simulink library "mpc555drivers"  (Simulink 6.0)
settings: Solver=ode45  SolverMode=SingleTasking  StartTime=0.0  StopTime=10.0  RelTol=1e-3
PreLoadFcn:
  | RTWConfigurationCB('preloadfcn', bdroot);
InitFcn:
  | % START RTW CONFIGURATION CODE %
  | RTWConfigurationCB('rtw_target_initfcn',gcs);
  | % END RTW CONFIGURATION CODE %
undefined symbols (not defined in the file or in its folder): pmax, scale
libraries: passthrough x52, driver_interface_library x18, mpc555toucan x11, mpc555extras x9, config_library x7, exprofilelib x4, simulink x3, mpc555drivers x2, canblocks x1
(part 2 of 3)

== system mpc555drivers/Time Processor Unit (TPU3) ==
  Subsystem Resource Configuration Class : config_library/Subsystem Resource Configuration Class  Tag=CONFIGURATION DATA CLASS  dClassName=MPC555dkConfig.TPU  rClassName=MPC555dkConfig.TPU_RESOURCES
  TPU3 Digital In : Subsystem  PropExecContextAcrossSSBoundary=on  mask(MPC555 Digital Input (TPU3)){module=A, channel=0, channel_priority=Medium, sampleTime=0.1, enablePassThru=off}
      mask prompts: module "TPU module:"; channel "TPU channel number:"; channel_priority "Channel priority:"; sampleTime "Sample time:"; enablePassThru "Enable pass through (show simulation input)"
      mask help: Configures a Time Processor Unit (TPU3) channel for digital input. Reads the logical state of the specified TPU channel pin.
      mask init:
      | simulinkPortControl(gcbh,'enable','PassThrough',enablePassThru);
      | 
      | %Deprecation warning for passthrough
      | if (enablePassThru)
      | 	passThroughDeprecationWarning;
      | end;
      | 
      | % decrement the channel to map from 0..15
      | channel = channel - 1;
      | 
      | % verify module selection
      | mpc5xx_tpu_verify_modules(gcb);
      | 
      | % Perform Resource Configuration
      | type = ['TPU_' module '_CHANNELS'];
      | RTWConfiguration.Target.acquireResourceForBlock(      ...
      |    gcb,                    ...   % Current block
      |    'MPC555dkConfig.TPU', ...   % Configuration Class
      |    type,          ...   % Resource Type associated with the configuration class
      |    num2str(channel),                    ...   % Resource being requested
      |    'TPU Channel'            ...   % Lable to be used in error messages
      | );
      mask Help: helpview([docroot '/toolbox/mpc555dk/mpc555dk.map'], 'TPU_Dig_In');
      mask StyleString: popup(A|B|C),popup(0|1|2|3|4|5|6|7|8|9|10|11|12|13|14|15),popup(Low|Medium|High),edit,checkbox
      mask Display: disp(['Digital In\n(TPU3)']);
  TPU3 Digital Out : Subsystem  PropExecContextAcrossSSBoundary=on  mask(MPC555 Digital Output (TPU3)){module=A, channel=0, channel_priority=Medium, sampleTime=-1, enablePassThru=off}
      mask prompts: module "TPU module:"; channel "TPU channel number:"; channel_priority "Channel priority:"; sampleTime "Sample time:"; enablePassThru "Enable pass through (show simulation output)"
      mask help: Configures a Time Processor Unit (TPU3) channel for digital output. When the input signal is greater than zero a logical one is written to the corresponding pin; otherwise a logical zero is written.
      mask init:
      | simulinkPortControl(gcbh,'enable','PassThrough',enablePassThru);
      | 
      | %Deprecation warning for passthrough
      | if (enablePassThru)
      | 	passThroughDeprecationWarning;
      | end;
      | 
      | % decrement the channel to map from 0..15
      | channel = channel - 1;
      | 
      | % verify module selection
      | mpc5xx_tpu_verify_modules(gcb);
      | 
      | % Perform Resource Configuration
      | type = ['TPU_' module '_CHANNELS'];
      | RTWConfiguration.Target.acquireResourceForBlock(      ...
      |    gcb,                    ...   % Current block
      |    'MPC555dkConfig.TPU', ...   % Configuration Class
      |    type,          ...   % Resource Type associated with the configuration class
      |    num2str(channel),                    ...   % Resource being requested
      |    'TPU Channel'            ...   % Lable to be used in error messages
      | );
      mask Help: helpview([docroot '/toolbox/mpc555dk/mpc555dk.map'], 'TPU_Dig_Out');
      mask StyleString: popup(A|B|C),popup(0|1|2|3|4|5|6|7|8|9|10|11|12|13|14|15),popup(Low|Medium|High),edit,checkbox
      mask Display: disp(['Digital Out\n (TPU3)'])
  TPU3 Fast Quadrature Decode : Subsystem  PropExecContextAcrossSSBoundary=on  mask(MPC555 Fast Quadrature Decode (TPU3)){module=A, channel=0 and 1, channel_priority=Medium, fast_mode=off, init_position_count=0, pc_alias=, sampleTime=0.1, enablePassThru=off}
      mask prompts: module "TPU module:"; channel "TPU channel numbers (primary and secondary):"; channel_priority "Channel priority:"; fast_mode "Show Fast Mode port"; init_position_count "Initial value for POSITION_COUNT:"; pc_alias "POSITION_COUNT parameter alias (optional):"; sampleTime "Sample time:"; enablePassThru "Enable pass through (show simulation input)"
      mask help:
      | Configures a pair of Time Processor Unit (TPU3) channels for Fast Quadrature Decode (FQD).   Decodes a pair of out-of-phase input signals in order to increment or decrement the position counter (block output).
      |
      | The POSITION_COUNT parameter can be made available easily to other TPU blocks such as the NITC function by providing an alias.
      mask init:
      | % enable / disable ports according to mask selections
      | simulinkPortControl(gcbh, 'enable', 'FastMode', fast_mode);
      | simulinkPortControl(gcbh, 'enable', 'PassThrough', enablePassThru);
      | 
      | %Deprecation warning for passthrough
      | if (enablePassThru)
      | 	passThroughDeprecationWarning;
      | end;
      | 
      | % decrement the channel to map from 0..15
      | channel = channel - 1;
      | % resource allocation for the primary channel + secondary channel
      | % mpc555_tpu_fqd_validate acquires resouce for primary channel, and
      | % primary channel + 1 (secondary channel)
      | % Perform Resource Configuration
      | type = ['TPU_' module '_CHANNELS'];
      | 
      | % verify module selection
      | mpc5xx_tpu_verify_modules(gcb);
      | 
      | RTWConfiguration.Target.acquireResourceForBlock(      ...
      |    gcb,                    ...   % Current block
      |    'MPC555dkConfig.TPU', ...   % Configuration Class
      |    type,          ...   % Resource Type associated with the configuration class
      |    { num2str(channel) num2str(channel+1) },                    ...   % Resource being requested
      |    'TPU Channel'            ...   % Lable to be used in error messages
      | );
      | 
      | % make sure the variables are consistent
      | % we cannot just rely on the mask callbacks!
      | mpc555_tpu_fqd_config('model_initialisation', gcb, init_position_count);
      mask Help: helpview([docroot '/toolbox/mpc555dk/mpc555dk.map'], 'TPU_Fast_Quad_Decode');
      mask StyleString: popup(A|B|C),popup(0 and 1|1 and 2|2 and 3|3 and 4|4 and 5|5 and 6|6 and 7|7 and 8|8 and 9|9 and 10|10 and 11|11 and 12|12 and 13|13 and 14|14 and 15),popup(Low|Medium|High),checkbox,edit,edit,edit,checkbox
      mask CallbackString: ||||mpc555_tpu_fqd_config('initPositionCallback', gcbh);|||
      mask Display: disp(sprintf('FQD\n(TPU3)'));
  TPU3 New Input Capture/ Input Transition Counter : Subsystem  PropExecContextAcrossSSBoundary=on  mask(MPC555 New Input Capture/Input Transition Counter (TPU3)){module=A, channel=0, channel_priority=Medium, finalTransTime=on, transCount=off, lastTransTime=off, transitionType=Rising Edge, captureType=TCR1 Value, parameterLocation=Channel and Parameter Index, captureChannel=0, captureParam=0, captureParamAlias=, maxCount=1, sampleTime=0.1, enablePassThru=off}
      mask prompts: module "TPU module:"; channel "TPU channel number:"; channel_priority "Channel priority:"; finalTransTime "Show FINAL_TRANS_TIME port"; transCount "Show TRANS_COUNT port"; lastTransTime "Show LAST_TRANS_TIME port"; transitionType "Detect transition on:"; captureType "Capture:"; parameterLocation "Specify parameter location by:"; captureChannel "TPU channel to capture parameter from:"; captureParam "Channel parameter (16-bit) to capture:"; captureParamAlias "Parameter alias:"; maxCount "Number of transitions before capture and reset (MAX_COUNT):"; sampleTime "Sample time:"; enablePassThru "Enable pass through  (show simulation input)"
      mask help: Configures a Time Processor Unit (TPU3) channel for New Input Capture/Input Transition Counter (NITC). Counts individual transitions on the input pin, and allows the capture of a TCR or TPU parameter RAM value after a selectable number of pin transitions.
      mask init:
      | % enable / disable ports according to mask selections
      | simulinkPortControl(gcbh, 'enable', 'FinalTransTime', finalTransTime);
      | simulinkPortControl(gcbh, 'enable', 'TransCount', transCount);
      | simulinkPortControl(gcbh, 'enable', 'LastTransTime', lastTransTime);
      | simulinkPortControl(gcbh, 'enable', 'PassThroughFinalTransTime', finalTransTime & enablePassThru);
      | simulinkPortControl(gcbh, 'enable', 'PassThroughTransCount', transCount & enablePassThru);
      | simulinkPortControl(gcbh, 'enable', 'PassThroughLastTransTime', lastTransTime & enablePassThru);
      | 
      | %Deprecation warning for passthrough
      | if (enablePassThru)
      | 	passThroughDeprecationWarning;
      | end;
      | 
      | % decrement the channel to map from 0..15
      | channel = channel - 1;
      | % decrement the capture channel to map from 0..15
      | captureChannel = captureChannel - 1;
      | % decrement the capture param to map from 0..7
      | captureParam = captureParam - 1;
      | 
      | % check the MAX_COUNT param at model update time
      | % as well as in the mask callback
      | mpc555_tpu_nitc_config('model_initialisation', gcb, maxCount);
      | 
      | % check the alias parameter is not empty
      | if captureType == 2 && parameterLocation == 2
      | 	captureParamAlias = strtrim(captureParamAlias);
      | 	if isempty(captureParamAlias)
      | 		error(sprintf('\n"Named parameter to be captured" parameter cannot be empty'));
      | 	end
      | end
      | 
      | % verify module selection
      | mpc5xx_tpu_verify_modules(gcb);
      | 
      | % Perform Resource Configuration
      | type = ['TPU_' module '_CHANNELS'];
      | RTWConfiguration.Target.acquireResourceForBlock(      ...
      |    gcb,                    ...   % Current block
      |    'MPC555dkConfig.TPU', ...   % Configuration Class
      |    type,          ...   % Resource Type associated with the configuration class
      |    num2str(channel),                    ...   % Resource being requested
      |    'TPU Channel'            ...   % Lable to be used in error messages
      | );
      mask Help: helpview([docroot '/toolbox/mpc555dk/mpc555dk.map'], 'TPU_NITC');
      mask StyleString: popup(A|B|C),popup(0|1|2|3|4|5|6|7|8|9|10|11|12|13|14|15),popup(Low|Medium|High),checkbox,checkbox,checkbox,popup(Rising Edge|Falling Edge|Either Edge),popup(TCR1 Value|Parameter RAM Value),popup(Channel and Parameter Index|Parameter Alias),popup(0|1|2|3|4|5|6|7|8|9|10|11|12|13|14|15),popup(0|1|2|3|4|5|6|7),edit,edit,edit,checkbox
      mask CallbackString:
      | |||||||switch get_param(gcb,'captureType')
      | 	case 'TCR1 Value'
      | 	    simUtil_maskParam('disable', gcb, 'parameterLocation');
      | 	case 'Parameter RAM Value'
      | 		simUtil_maskParam('enable', gcb, 'parameterLocation');
      | end
      | simUtil_maskParam('execcallback', gcb, 'parameterLocation');|if simUtil_maskParam('isenable', gcb, 'parameterLocation')
      | 	switch get_param(gcb,'parameterLocation')
      | 	case 'Channel and Parameter Index'
      | 	    simUtil_maskParam('enable', gcb, 'captureChannel');
      | 		simUtil_maskParam('enable', gcb, 'captureParam');
      | 		simUtil_maskParam('disable', gcb, 'captureParamAlias');
      | 
      | 	case 'Parameter Alias'
      | 		simUtil_maskParam('disable', gcb, 'captureChannel');
      | 		simUtil_maskParam('disable', gcb, 'captureParam');
      | 		simUtil_maskParam('enable', gcb, 'captureParamAlias');
      | 	end
      | else
      | 		simUtil_maskParam('disable', gcb, 'captureChannel');
      | 		simUtil_maskParam('disable', gcb, 'captureParam');
      | 		simUtil_maskParam('disable', gcb, 'captureParamAlias');
      | end||||mpc555_tpu_nitc_config('max_count_callback', gcb);||
      mask Display: disp(['NITC\n(TPU3)']);
  TPU3 Programmable Time Accumulator : Subsystem  PropExecContextAcrossSSBoundary=on  mask(MPC555 Programmable Time Accumulator (TPU3)){module=A, channel=0, channel_priority=Medium, timeAccum=on, periodCount=off, mode=Total high time, maxCount=1, sampleTime=0.1, enablePassThru=off}
      mask prompts: module "TPU module:"; channel "TPU channel number:"; channel_priority "Channel priority:"; timeAccum "Show time accumulation (32-bit) port"; periodCount "Show PERIOD_COUNT port"; mode "Measure:"; maxCount "Number of periods to measure over (MAX_COUNT):"; sampleTime "Sample time:"; enablePassThru "Enable pass through (show simulation input)"
      mask help: Configures a Time Processor Unit (TPU3) channel for Programmable Time Accumulator (PTA). Measures high time, low time or total period over a selectable number of periods on the input pin.
      mask init:
      | % enable / disable ports according to mask selections
      | simulinkPortControl(gcbh, 'enable', 'TimeAccum', timeAccum);
      | simulinkPortControl(gcbh, 'enable', 'PeriodCount', periodCount);
      | simulinkPortControl(gcbh, 'enable', 'PassThroughTimeAccum', timeAccum & enablePassThru);
      | simulinkPortControl(gcbh, 'enable', 'PassThroughPeriodCount', periodCount & enablePassThru);
      | 
      | %Deprecation warning for passthrough
      | if (enablePassThru)
      | 	passThroughDeprecationWarning;
      | end;
      | 
      | % decrement the channel to map from 0..15
      | channel = channel - 1;
      | 
      | % check the MAX_COUNT param at model update time
      | % as well as in the mask callback
      | mpc555_tpu_pta_config('model_initialisation', gcb, maxCount);
      | 
      | % verify module selection
      | mpc5xx_tpu_verify_modules(gcb);
      | 
      | % Perform Resource Configuration
      | type = ['TPU_' module '_CHANNELS'];
      | RTWConfiguration.Target.acquireResourceForBlock(      ...
      |    gcb,                    ...   % Current block
      |    'MPC555dkConfig.TPU', ...   % Configuration Class
      |    type,          ...   % Resource Type associated with the configuration class
      |    num2str(channel),                    ...   % Resource being requested
      |    'TPU Channel'            ...   % Lable to be used in error messages
      | );
      mask Help: helpview([docroot '/toolbox/mpc555dk/mpc555dk.map'], 'TPU_PTA');
      mask StyleString: popup(A|B|C),popup(0|1|2|3|4|5|6|7|8|9|10|11|12|13|14|15),popup(Low|Medium|High),checkbox,checkbox,popup(Total high time|Total low time|Total period (start on rising edge)|Total period (start on falling edge)),edit,edit,checkbox
      mask CallbackString: ||||||mpc555_tpu_pta_config('max_count_callback', gcb);||
      mask Display: disp(['PTA\n(TPU3)']);
  TPU3 Pulse Width Modulation Out : Subsystem  PropExecContextAcrossSSBoundary=on  mask(MPC555 Pulse Width Modulation Output (TPU3)){module=A, channel=0, channel_priority=Medium, block_period=off, timing_settings=off, ideal_period=0.02, PWMPER=12500, actual_period=0.02, sampleTime=-1, enablePassThru=off}
      mask prompts: module "TPU module:"; channel "TPU channel number:"; channel_priority "Channel priority:"; block_period "Use input port for pulse period register value"; timing_settings "Edit period register manually"; ideal_period "Waveform ideal period:"; PWMPER "Pulse period register (PWMPER):"; actual_period "Waveform actual period:"; sampleTime "Sample time:"; enablePassThru "Enable pass through (show simulation output)"
      mask help: Configures a Time Processor Unit (TPU3) channel for pulse width modulation (PWM) output. An input signal in the range 0 to 1 generates a PWM output with corresponding duty cycle; input signals above (below) this range cause the duty cycle to saturate at 100% (0%).
      mask init:
      | % enable / disable ports according to mask selections
      | simulinkPortControl(gcbh, 'enable', 'Period', block_period);
      | simulinkPortControl(gcbh, 'enable', 'PassThroughDutyCycle', enablePassThru);
      | simulinkPortControl(gcbh, 'enable', 'PassThroughPeriod', enablePassThru & block_period);
      | 
      | %Deprecation warning for passthrough
      | if (enablePassThru)
      | 	passThroughDeprecationWarning;
      | end;
      | 
      | % decrement the channel to map from 0..15
      | channel = channel - 1;
      | 
      | % verify module selection
      | mpc5xx_tpu_verify_modules(gcb);
      | 
      | % Perform Resource Configuration
      | type = ['TPU_' module '_CHANNELS'];
      | RTWConfiguration.Target.acquireResourceForBlock(      ...
      |    gcb,                    ...   % Current block
      |    'MPC555dkConfig.TPU', ...   % Configuration Class
      |    type,          ...   % Resource Type associated with the configuration class
      |    num2str(channel),                    ...   % Resource being requested
      |    'TPU Channel'            ...   % Lable to be used in error messages
      | );
      | 
      | % make sure the variables are consistent
      | % we cannot just rely on the mask callbacks!
      | PWMPER = mpc555_tpu_pwm_config('model_initialisation',gcb, PWMPER, ideal_period);
      mask Help: helpview([docroot '/toolbox/mpc555dk/mpc555dk.map'], 'TPU_PWM_Out');
      mask StyleString: popup(A|B|C),popup(0|1|2|3|4|5|6|7|8|9|10|11|12|13|14|15),popup(Low|Medium|High),checkbox,checkbox,edit,edit,edit,edit,checkbox
      mask CallbackString: |||mpc555_tpu_pwm_config('block_period_callback',gcb);|mpc555_tpu_pwm_config('timing_settings_callback',gcb);|mpc555_tpu_pwm_config('ideal_period_callback',gcb);|mpc555_tpu_pwm_config('PWMPER_callback',gcb);|||
      mask Display: disp(sprintf('PWM Out\n(TPU3)'))

== system mpc555drivers/Watchdog ==
  Initialize Watchdog : mpc555extras/Custom Code  unique=Generate for every instance  key='_WATCHDOG_'  location=Model Start Function  top=''  middle=''  bottom=model_init_function_code

== system mpc555drivers/Enhanced Queued Analog-To-Digital Converter Module-64/QADCE Analog In ==
  note: NOTE: Data direction register has 0 reset value
      | ->
      | all pins configured for input
  Extended Custom Code : driver_interface_library/Custom Code
  RTW memory get : driver_interface_library/Input Driver  t=t  expr=register  portWidth=length(channels)  pOpt=[]  expression_type=Expression
  Subsystem : Subsystem  PropExecContextAcrossSSBoundary=on  mask{type=outDType}
      mask prompts: type "Data Type"
      mask init:
      | block = find_system(gcb,'followlinks','on','lookundermasks','on','tag','type_block');
      | set_param(block{1},'DataType',type);
  Out : Outport
  wires:
  Subsystem/1(Out1) -> Out/1
  RTW memory get/1 -> Subsystem/1(In1)

== system mpc555drivers/Enhanced Queued Analog-To-Digital Converter Module-64/QADCE Digital In ==
  note: NOTE: Data direction register has 0 reset value
      | ->
      | all pins configured for input
  Bitwise Operator1 : mpc555extras/Bitwise Operator  logicop=AND  zeroTest=Test If Not Zero  UseBitMask=on  BitMask=masks  maskInBinary=off
  Data Type Conversion : DataTypeConversion  OutDataTypeMode=boolean  SaturateOnIntegerOverflow=on  RndMeth=Zero
  RTW memory get : driver_interface_library/Input Driver  t=t  expr=register  portWidth=1  pOpt=[]  expression_type=Expression
  Signal Specification : SignalSpecification  DataType=uint8
  Out : Outport
  wires:
  Data Type Conversion/1 -> Out/1
  Signal Specification/1 -> Bitwise Operator1/1
  RTW memory get/1 -> Signal Specification/1
  Bitwise Operator1/1 -> Data Type Conversion/1

== system mpc555drivers/Execution Profiling/MPC555 Execution Profiling via CAN A ==
  Execution Profiling Output Data1 : exprofilelib/Execution Profiling Output Data  t=t
  Send data over CAN : Subsystem  TreatAsAtomicUnit=on  PropExecContextAcrossSSBoundary=on
  Start execution profiling : Subsystem  PropExecContextAcrossSSBoundary=on
  Terminator : Terminator
  TouCAN Receive : mpc555toucan/TouCAN Receive  module=A  ids=commandId  notification_type=Function Call Outport  auto_select_buffer=on  bufferids=14  use_queue=off  queue_length=3  message_type=Extended (29-bit identifier)  t=t
  wires:
  Execution Profiling Output Data1/2 -> Send data over CAN/1(In1)
  Execution Profiling Output Data1/1 -> Send data over CAN/Enable
  TouCAN Receive/1 -> Start execution profiling/Trigger
  TouCAN Receive/2 -> Terminator/1

== system mpc555drivers/Execution Profiling/MPC555 Execution Profiling via SCI1 ==
  Constant : Constant  OutDataTypeMode=uint32
  Send Execution Profiling Data via Serial : Subsystem  PropExecContextAcrossSSBoundary=on
  Serial Receive : mpc555drivers/Serial Communications Interface (SCI)/Serial Receive  module=1  show_length=on  max_length=1  show_reset=off  show_bytes_read=on  show_flags=off  show_overrun=off  T=t
  Serial Transmit Status : S-Function  FunctionName=qsmcm_sci_status  Parameters=T, module  mask(SCI Status){module=1, T=t}
      mask prompts: module "SCI module:"; T "Sample time:"
      mask help: Read data from the QSMCM SCI status register. In particular, the Transmission Complete flag TC is equal to 0 if a transmission is in progress, or 1 if any transmission is complete.
      mask init:
      | % check for a Resource Config block, and make sure it is MPC555
      | target = RTWConfigurationCB('get_target', gcb);
      | target.checkName('MPC555');
      mask StyleString: popup(1|2),edit
      mask Display: text(0.5, 0.5, ['SCI' num2str(module) '\nStatus'],'horizontalAlignment','center'); port_label('input',1,'Data'); port_label('output', 1, 'TC');
  Start Profiling : Subsystem  PropExecContextAcrossSSBoundary=on
  wires:
  Serial Transmit Status/1 -> Send Execution Profiling Data via Serial/Enable
  Constant/1 -> Serial Receive/1
  Serial Receive/1 -> Start Profiling/1(Data In)
  Serial Receive/2 -> Start Profiling/Enable  "num bytes received"

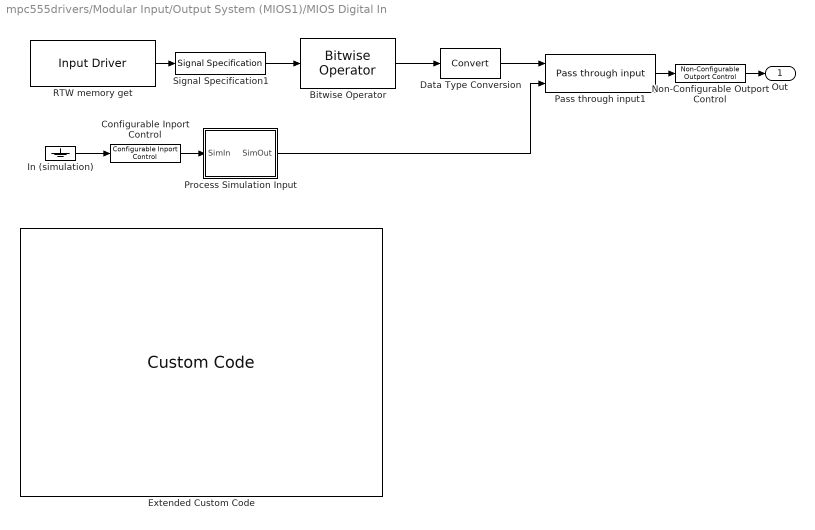
== system mpc555drivers/Modular Input/Output System (MIOS1)/MIOS Digital In ==
  Bitwise Operator : mpc555extras/Bitwise Operator  logicop=AND  zeroTest=No Test  UseBitMask=on  BitMask=masks  maskInBinary=on
  Configurable Inport Control : passthrough/Configurable Inport Control  portNum=1  portName=PassThrough  isEnabled=0  isConfigurable=1  isInport=1
  Data Type Conversion : DataTypeConversion  OutDataTypeMode=boolean  SaturateOnIntegerOverflow=on  RndMeth=Zero
  Extended Custom Code : driver_interface_library/Custom Code
  In (simulation) : Ground
  Non-Configurable Outport Control : passthrough/Non-Configurable Outport Control  portNum=1  isEnabled=1  isConfigurable=0  isInport=0
  Pass through input1 : passthrough/Pass through input
  Process Simulation Input : Subsystem  PropExecContextAcrossSSBoundary=on
  RTW memory get : driver_interface_library/Input Driver  t=t  expr='MIOS1.MPIOSM32DR.R'  portWidth=1  pOpt=[]  expression_type=Not expression
  Signal Specification1 : SignalSpecification  DataType=uint16
  Out : Outport
  wires:
  Pass through input1/1 -> Non-Configurable Outport Control/1
  RTW memory get/1 -> Signal Specification1/1
  In (simulation)/1 -> Configurable Inport Control/1
  Process Simulation Input/1(SimOut) -> Pass through input1/2
  Signal Specification1/1 -> Bitwise Operator/1
  Bitwise Operator/1 -> Data Type Conversion/1
  Data Type Conversion/1 -> Pass through input1/1
  Configurable Inport Control/1 -> Process Simulation Input/1(SimIn)
  Non-Configurable Outport Control/1 -> Out/1

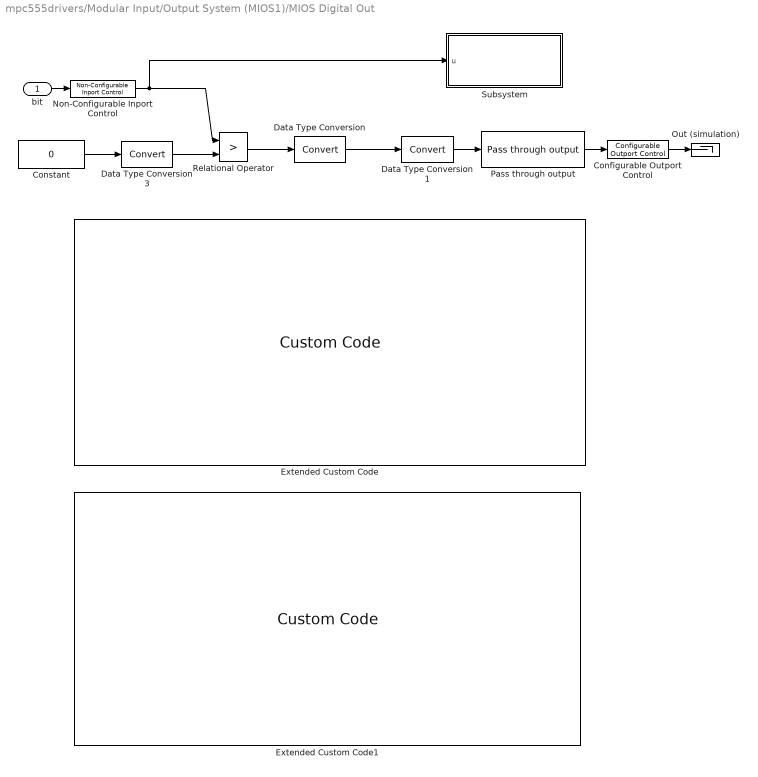
== system mpc555drivers/Modular Input/Output System (MIOS1)/MIOS Digital Out ==
  bit : Inport  Port=1  SampleTime=t  LatchInput=off
  Configurable Outport Control : passthrough/Configurable Outport Control  portNum=1  portName=PassThrough  isEnabled=0  isConfigurable=1  isInport=0
  Constant : Constant  Value=0
  Data Type Conversion : DataTypeConversion  OutDataTypeMode=boolean  SaturateOnIntegerOverflow=on  RndMeth=Zero
  Data Type Conversion1 : DataTypeConversion  SaturateOnIntegerOverflow=on  RndMeth=Zero
  Data Type Conversion3 : DataTypeConversion  SaturateOnIntegerOverflow=on  RndMeth=Zero
  Extended Custom Code : driver_interface_library/Custom Code
  Extended Custom Code1 : driver_interface_library/Custom Code
  Non-Configurable Inport Control : passthrough/Non-Configurable Inport Control  portNum=1  isEnabled=1  isConfigurable=0  isInport=1
  Out (simulation) : Terminator
  Pass through output : passthrough/Pass through output  driverBlock=gcs
  Relational Operator : RelationalOperator  Operator=>  InputSameDT=on
  Subsystem : Subsystem  TreatAsAtomicUnit=on  PropExecContextAcrossSSBoundary=on
  wires:
  bit/1 -> Non-Configurable Inport Control/1
  Relational Operator/1 -> Data Type Conversion/1
  Constant/1 -> Data Type Conversion3/1
  Data Type Conversion/1 -> Data Type Conversion1/1
  Pass through output/1 -> Configurable Outport Control/1
  Data Type Conversion1/1 -> Pass through output/1
  Data Type Conversion3/1 -> Relational Operator/2
  Non-Configurable Inport Control/1 -> Relational Operator/1, Subsystem/1(u)
  Configurable Outport Control/1 -> Out (simulation)/1

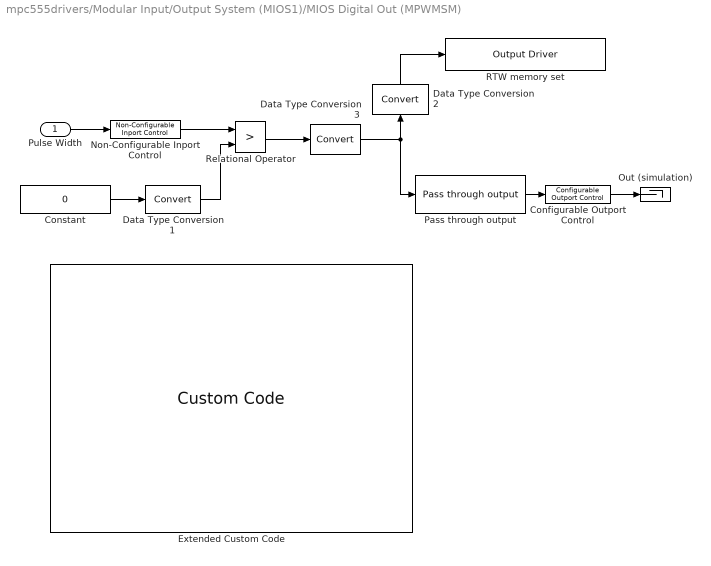
== system mpc555drivers/Modular Input/Output System (MIOS1)/MIOS Digital Out (MPWMSM) ==
  Pulse Width : Inport  Port=1  LatchInput=off
  Configurable Outport Control : passthrough/Configurable Outport Control  portNum=1  portName=PassThrough  isEnabled=0  isConfigurable=1  isInport=0
  Constant : Constant  Value=0
  Data Type Conversion1 : DataTypeConversion  SaturateOnIntegerOverflow=on  RndMeth=Zero
  Data Type Conversion2 : DataTypeConversion  Orientation=up  OutDataTypeMode=uint16  SaturateOnIntegerOverflow=on  RndMeth=Zero
  Data Type Conversion3 : DataTypeConversion  SaturateOnIntegerOverflow=on  RndMeth=Zero
  Extended Custom Code : driver_interface_library/Custom Code
  Non-Configurable Inport Control : passthrough/Non-Configurable Inport Control  portNum=1  isEnabled=1  isConfigurable=0  isInport=1
  Out (simulation) : Terminator
  Pass through output : passthrough/Pass through output  driverBlock=gcs
  RTW memory set : driver_interface_library/Output Driver  operation_type=LHS Assignment  input_is_contiguous=off  t=t  expr=[ 'MIOS1.MPWMSM' module 'SCR.B.POL']  port_width=1  pOpt=[]
  Relational Operator : RelationalOperator  Operator=>  InputSameDT=on
  wires:
  Pass through output/1 -> Configurable Outport Control/1
  Pulse Width/1 -> Non-Configurable Inport Control/1
  Relational Operator/1 -> Data Type Conversion3/1
  Constant/1 -> Data Type Conversion1/1
  Data Type Conversion1/1 -> Relational Operator/2
  Data Type Conversion2/1 -> RTW memory set/1
  Data Type Conversion3/1 -> Data Type Conversion2/1, Pass through output/1
  Non-Configurable Inport Control/1 -> Relational Operator/1
  Configurable Outport Control/1 -> Out (simulation)/1

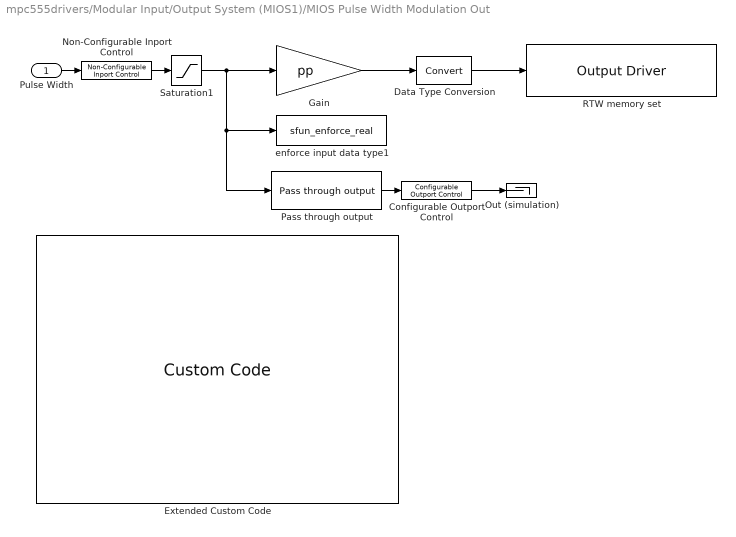
== system mpc555drivers/Modular Input/Output System (MIOS1)/MIOS Pulse Width Modulation Out ==
  Pulse Width : Inport  Port=1  SampleTime=t  LatchInput=off
  Configurable Outport Control : passthrough/Configurable Outport Control  portNum=1  portName=PassThrough  isEnabled=0  isConfigurable=1  isInport=0
  Data Type Conversion : DataTypeConversion  OutDataTypeMode=uint16  RndMeth=Zero
  Extended Custom Code : driver_interface_library/Custom Code
  Gain : Gain  Gain=pp  SaturateOnIntegerOverflow=on
  Non-Configurable Inport Control : passthrough/Non-Configurable Inport Control  portNum=1  isEnabled=1  isConfigurable=0  isInport=1
  Out (simulation) : Terminator
  Pass through output : passthrough/Pass through output  driverBlock=gcs
  RTW memory set : driver_interface_library/Output Driver  operation_type=LHS Assignment  input_is_contiguous=off  t=t  expr=['MIOS1.MPWMSM' num2str(module) 'PULR.R' ]  port_width=1  pOpt=[]
  Saturation1 : Saturate  UpperLimit=1  LowerLimit=0  ZeroCross=off
  enforce input data type1 : S-Function  FunctionName=sfun_enforce_real
  wires:
  Pass through output/1 -> Configurable Outport Control/1
  Gain/1 -> Data Type Conversion/1
  Data Type Conversion/1 -> RTW memory set/1
  Pulse Width/1 -> Non-Configurable Inport Control/1
  Non-Configurable Inport Control/1 -> Saturation1/1
  Configurable Outport Control/1 -> Out (simulation)/1
  Saturation1/1 -> enforce input data type1/1, Pass through output/1, Gain/1

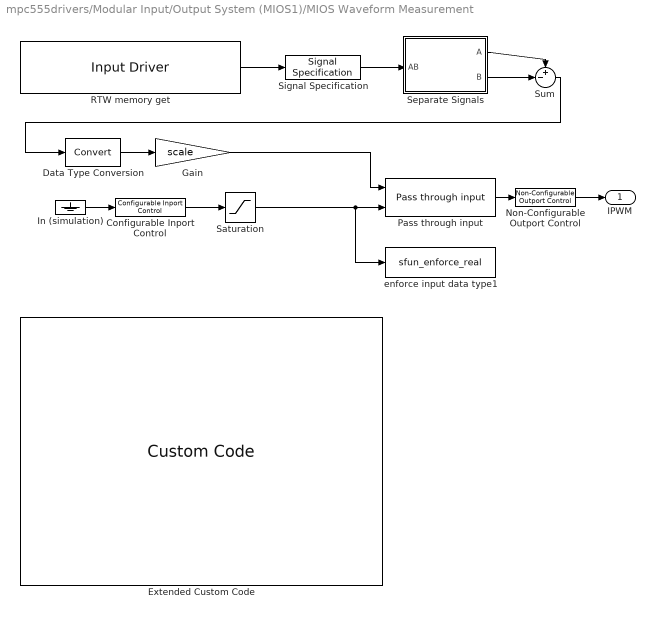
== system mpc555drivers/Modular Input/Output System (MIOS1)/MIOS Waveform Measurement ==
  Configurable Inport Control : passthrough/Configurable Inport Control  portNum=1  portName=PassThrough  isEnabled=0  isConfigurable=1  isInport=1
  Data Type Conversion : DataTypeConversion  SaturateOnIntegerOverflow=on  RndMeth=Zero
  Extended Custom Code : driver_interface_library/Custom Code
  Gain : Gain  Gain=scale  SaturateOnIntegerOverflow=on
  In (simulation) : Ground
  Non-Configurable Outport Control : passthrough/Non-Configurable Outport Control  portNum=1  isEnabled=1  isConfigurable=0  isInport=0
  Pass through input : passthrough/Pass through input
  RTW memory get : driver_interface_library/Input Driver  t=t  expr=['*((uint32_T *)&(MIOS1.MDASM' num2str(module) 'AR.R))']  portWidth=1  pOpt=[]  expression_type=Expression
  Saturation : Saturate  UpperLimit=pmax  LowerLimit=0  ZeroCross=off
  Separate Signals : Subsystem  PropExecContextAcrossSSBoundary=on
  Signal Specification : SignalSpecification  DataType=uint32
  Sum : Sum  Inputs=+-|  InputSameDT=on
  enforce input data type1 : S-Function  FunctionName=sfun_enforce_real
  IPWM : Outport
  wires:
  Gain/1 -> Pass through input/1
  In (simulation)/1 -> Configurable Inport Control/1
  Pass through input/1 -> Non-Configurable Outport Control/1
  Separate Signals/2(B) -> Sum/2
  Separate Signals/1(A) -> Sum/1
  Signal Specification/1 -> Separate Signals/1(AB)
  Data Type Conversion/1 -> Gain/1
  RTW memory get/1 -> Signal Specification/1
  Sum/1 -> Data Type Conversion/1
  Saturation/1 -> enforce input data type1/1, Pass through input/2
  Configurable Inport Control/1 -> Saturation/1
  Non-Configurable Outport Control/1 -> IPWM/1

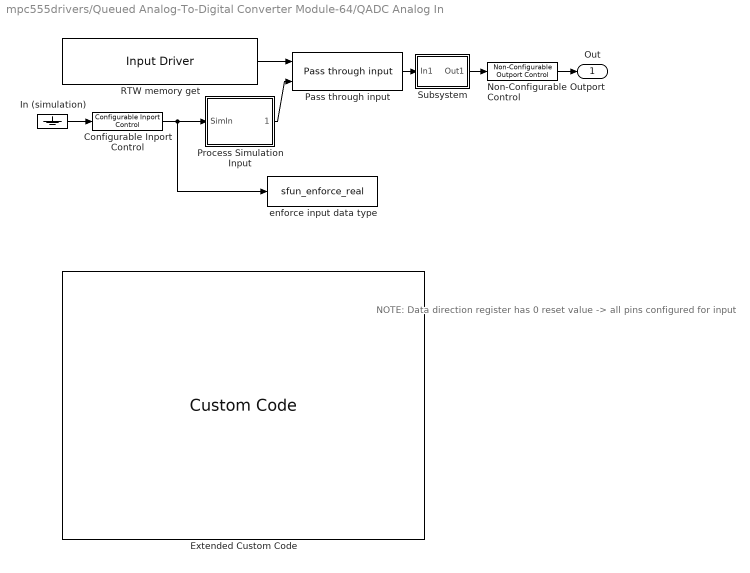
== system mpc555drivers/Queued Analog-To-Digital Converter Module-64/QADC Analog In ==
  note: NOTE: Data direction register has 0 reset value
      | ->
      | all pins configured for input
  Configurable Inport Control : passthrough/Configurable Inport Control  portNum=1  portName=PassThrough  isEnabled=0  isConfigurable=1  isInport=1
  Extended Custom Code : driver_interface_library/Custom Code
  In (simulation) : Ground
  Non-Configurable Outport Control : passthrough/Non-Configurable Outport Control  portNum=1  isEnabled=1  isConfigurable=0  isInport=0
  Pass through input : passthrough/Pass through input
  Process Simulation Input : Subsystem  PropExecContextAcrossSSBoundary=on
  RTW memory get : driver_interface_library/Input Driver  t=t  expr=register  portWidth=length(channels)  pOpt=[]  expression_type=Not expression
  Subsystem : Subsystem  PropExecContextAcrossSSBoundary=on  mask{type=outDType}
      mask prompts: type "Data Type"
      mask init:
      | block = find_system(gcb,'followlinks','on','lookundermasks','on','tag','type_block');
      | set_param(block{1},'DataType',type);
  enforce input data type : S-Function  FunctionName=sfun_enforce_real
  Out : Outport
  wires:
  Pass through input/1 -> Subsystem/1(In1)
  RTW memory get/1 -> Pass through input/1
  Subsystem/1(Out1) -> Non-Configurable Outport Control/1
  Process Simulation Input/1(SimOut) -> Pass through input/2
  Configurable Inport Control/1 -> Process Simulation Input/1(SimIn), enforce input data type/1
  Non-Configurable Outport Control/1 -> Out/1
  In (simulation)/1 -> Configurable Inport Control/1

== system mpc555drivers/Queued Analog-To-Digital Converter Module-64/QADC Digital In ==
  note: NOTE: Data direction register has 0 reset value
      | ->
      | all pins configured for input
  Bitwise Operator1 : mpc555extras/Bitwise Operator  logicop=AND  zeroTest=Test If Not Zero  UseBitMask=on  BitMask=masks  maskInBinary=off
  Configurable Inport Control : passthrough/Configurable Inport Control  portNum=1  portName=PassThrough  isEnabled=0  isConfigurable=1  isInport=1
  Data Type Conversion : DataTypeConversion  OutDataTypeMode=boolean  SaturateOnIntegerOverflow=on  RndMeth=Zero
  In (simulation) : Ground
  Non-Configurable Outport Control : passthrough/Non-Configurable Outport Control  portNum=1  isEnabled=1  isConfigurable=0  isInport=0
  Pass through input : passthrough/Pass through input
  Process Simulation Input : Subsystem  PropExecContextAcrossSSBoundary=on
  RTW memory get : driver_interface_library/Input Driver  t=t  expr=register  portWidth=1  pOpt=[]  expression_type=Expression
  Signal Specification : SignalSpecification  DataType=uint8
  Out : Outport
  wires:
  Pass through input/1 -> Non-Configurable Outport Control/1
  Bitwise Operator1/1 -> Data Type Conversion/1
  RTW memory get/1 -> Signal Specification/1
  Signal Specification/1 -> Bitwise Operator1/1
  In (simulation)/1 -> Configurable Inport Control/1
  Process Simulation Input/1(SimOut) -> Pass through input/2
  Data Type Conversion/1 -> Pass through input/1
  Configurable Inport Control/1 -> Process Simulation Input/1(SimIn)
  Non-Configurable Outport Control/1 -> Out/1

== system mpc555drivers/Time Processor Unit (TPU3)/TPU3 Digital In ==
  Configurable Inport Control : passthrough/Configurable Inport Control  portNum=1  portName=PassThrough  isEnabled=0  isConfigurable=1  isInport=1
  In (simulation) : Ground
  Non-Configurable Outport Control : passthrough/Non-Configurable Outport Control  portNum=1  isEnabled=1  isConfigurable=0  isInport=0
  Pass through input : passthrough/Pass through input
  Process Simulation Input : Subsystem  PropExecContextAcrossSSBoundary=on
  S-Function : S-Function  FunctionName=sfun_tpu3_dig_in  Parameters=sampleTime, module, uint8(channel), uint8(channel_priority)
  Out1 : Outport
  wires:
  Non-Configurable Outport Control/1 -> Out1/1
  Configurable Inport Control/1 -> Process Simulation Input/1(SimIn)
  S-Function/1 -> Pass through input/1
  Process Simulation Input/1(SimOut) -> Pass through input/2
  In (simulation)/1 -> Configurable Inport Control/1
  Pass through input/1 -> Non-Configurable Outport Control/1

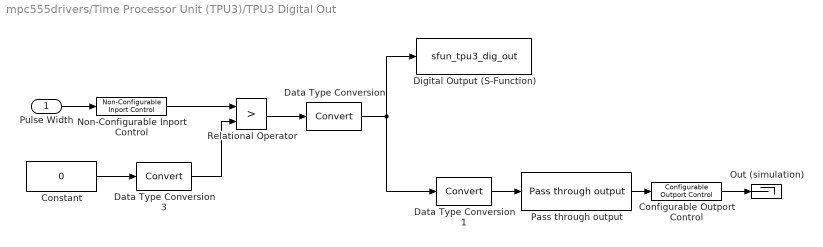
== system mpc555drivers/Time Processor Unit (TPU3)/TPU3 Digital Out ==
  Pulse Width : Inport  Port=1  LatchInput=off
  Configurable Outport Control : passthrough/Configurable Outport Control  portNum=1  portName=PassThrough  isEnabled=0  isConfigurable=1  isInport=0
  Constant : Constant  Value=0
  Data Type Conversion : DataTypeConversion  OutDataTypeMode=boolean  SaturateOnIntegerOverflow=on  RndMeth=Zero
  Data Type Conversion1 : DataTypeConversion  SaturateOnIntegerOverflow=on  RndMeth=Zero
  Data Type Conversion3 : DataTypeConversion  SaturateOnIntegerOverflow=on  RndMeth=Zero
  Digital Output (S-Function) : S-Function  FunctionName=sfun_tpu3_dig_out  Parameters=sampleTime, module, uint8(channel), uint8(channel_priority)
  Non-Configurable Inport Control : passthrough/Non-Configurable Inport Control  portNum=1  isEnabled=1  isConfigurable=0  isInport=1
  Out (simulation) : Terminator
  Pass through output : passthrough/Pass through output  driverBlock=gcs
  Relational Operator : RelationalOperator  Operator=>  InputSameDT=on
  wires:
  Configurable Outport Control/1 -> Out (simulation)/1
  Non-Configurable Inport Control/1 -> Relational Operator/1
  Pulse Width/1 -> Non-Configurable Inport Control/1
  Relational Operator/1 -> Data Type Conversion/1
  Constant/1 -> Data Type Conversion3/1
  Data Type Conversion/1 -> Digital Output (S-Function)/1, Data Type Conversion1/1
  Pass through output/1 -> Configurable Outport Control/1
  Data Type Conversion1/1 -> Pass through output/1
  Data Type Conversion3/1 -> Relational Operator/2

== system mpc555drivers/Time Processor Unit (TPU3)/TPU3 Fast Quadrature Decode ==
  Configurable Inport Control : passthrough/Configurable Inport Control  portNum=1  portName=FastMode  isEnabled=0  isConfigurable=1  isInport=1
  Configurable Inport Control1 : passthrough/Configurable Inport Control  portNum=2  portName=PassThrough  isEnabled=0  isConfigurable=1  isInport=1
  FQD Driver Code : S-Function  FunctionName=sfun_tpu3_fqd  Parameters=sampleTime, module, uint8(channel), uint8(channel_priority), uint16(init_position_count), fast_mode, pc_alias
  Non-Configurable Outport Control : passthrough/Non-Configurable Outport Control  portNum=1  isEnabled=1  isConfigurable=0  isInport=0
  Pass through input : passthrough/Pass through input
  Signal Specification : SignalSpecification  DataType=uint16
  fastMode : Ground
  positionCount Pass Through : Ground
  positionCount : Outport
  wires:
  FQD Driver Code/1 -> Pass through input/1
  Configurable Inport Control/1 -> FQD Driver Code/1
  Signal Specification/1 -> Pass through input/2
  Pass through input/1 -> Non-Configurable Outport Control/1
  Configurable Inport Control1/1 -> Signal Specification/1
  Non-Configurable Outport Control/1 -> positionCount/1
  fastMode/1 -> Configurable Inport Control/1
  positionCount Pass Through/1 -> Configurable Inport Control1/1

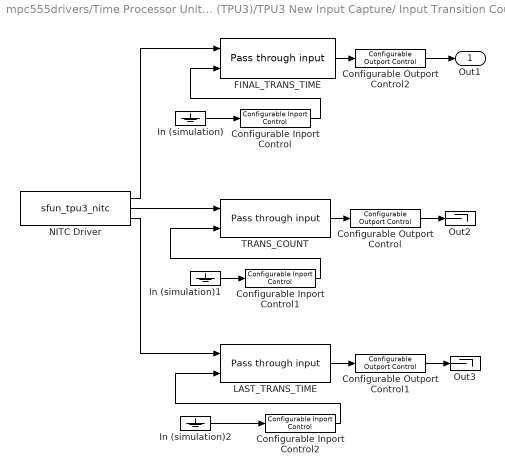
== system mpc555drivers/Time Processor Unit (TPU3)/TPU3 New Input Capture/ Input Transition Counter ==
  Configurable Inport Control : passthrough/Configurable Inport Control  portNum=1  portName=PassThroughFinalTransTime  isEnabled=0  isConfigurable=1  isInport=1
  Configurable Inport Control1 : passthrough/Configurable Inport Control  portNum=2  portName=PassThroughTransCount  isEnabled=0  isConfigurable=1  isInport=1
  Configurable Inport Control2 : passthrough/Configurable Inport Control  portNum=3  portName=PassThroughLastTransTime  isEnabled=0  isConfigurable=1  isInport=1
  Configurable Outport Control : passthrough/Configurable Outport Control  portNum=2  portName=TransCount  isEnabled=0  isConfigurable=1  isInport=0
  Configurable Outport Control1 : passthrough/Configurable Outport Control  portNum=3  portName=LastTransTime  isEnabled=0  isConfigurable=1  isInport=0
  Configurable Outport Control2 : passthrough/Configurable Outport Control  portNum=1  portName=FinalTransTime  isEnabled=1  isConfigurable=1  isInport=0
  FINAL_TRANS_TIME : passthrough/Pass through input
  In (simulation) : Ground
  In (simulation)1 : Ground
  In (simulation)2 : Ground
  LAST_TRANS_TIME : passthrough/Pass through input
  NITC Driver : S-Function  FunctionName=sfun_tpu3_nitc  Parameters=sampleTime, module, uint8(channel), uint8(channel_priority), uint8(transitionType), uint16(maxCount), uint8(captureType), uint8(parameterLocation), uint8(captureChannel), uint8(captureParam), uint8(transCount), uint8(lastTransTime), uint8(finalTransTime), captureParamAlias
  Out2 : Terminator
  Out3 : Terminator
  TRANS_COUNT : passthrough/Pass through input
  Out1 : Outport
  wires:
  NITC Driver/3 -> LAST_TRANS_TIME/1
  NITC Driver/2 -> TRANS_COUNT/1
  NITC Driver/1 -> FINAL_TRANS_TIME/1
  Configurable Outport Control1/1 -> Out3/1
  LAST_TRANS_TIME/1 -> Configurable Outport Control1/1
  In (simulation)2/1 -> Configurable Inport Control2/1
  Configurable Inport Control2/1 -> LAST_TRANS_TIME/2
  Configurable Outport Control/1 -> Out2/1
  TRANS_COUNT/1 -> Configurable Outport Control/1
  Configurable Inport Control1/1 -> TRANS_COUNT/2
  In (simulation)1/1 -> Configurable Inport Control1/1
  Configurable Outport Control2/1 -> Out1/1
  FINAL_TRANS_TIME/1 -> Configurable Outport Control2/1
  Configurable Inport Control/1 -> FINAL_TRANS_TIME/2
  In (simulation)/1 -> Configurable Inport Control/1

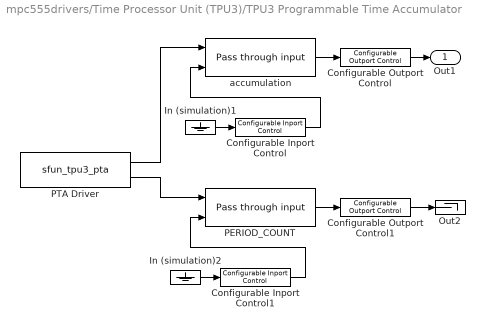
== system mpc555drivers/Time Processor Unit (TPU3)/TPU3 Programmable Time Accumulator ==
  Configurable Inport Control : passthrough/Configurable Inport Control  portNum=1  portName=PassThroughTimeAccum  isEnabled=0  isConfigurable=1  isInport=1
  Configurable Inport Control1 : passthrough/Configurable Inport Control  portNum=2  portName=PassThroughPeriodCount  isEnabled=0  isConfigurable=1  isInport=1
  Configurable Outport Control : passthrough/Configurable Outport Control  portNum=1  portName=TimeAccum  isEnabled=1  isConfigurable=1  isInport=0
  Configurable Outport Control1 : passthrough/Configurable Outport Control  portNum=2  portName=PeriodCount  isEnabled=0  isConfigurable=1  isInport=0
  In (simulation)1 : Ground
  In (simulation)2 : Ground
  Out2 : Terminator
  PERIOD_COUNT : passthrough/Pass through input
  PTA Driver : S-Function  FunctionName=sfun_tpu3_pta  Parameters=sampleTime, module, uint8(channel), uint8(channel_priority), uint8(mode), uint8(maxCount), uint8(timeAccum), uint8(periodCount)
  accumulation : passthrough/Pass through input
  Out1 : Outport
  wires:
  In (simulation)2/1 -> Configurable Inport Control1/1
  In (simulation)1/1 -> Configurable Inport Control/1
  Configurable Inport Control1/1 -> PERIOD_COUNT/2
  Configurable Inport Control/1 -> accumulation/2
  Configurable Outport Control1/1 -> Out2/1
  PERIOD_COUNT/1 -> Configurable Outport Control1/1
  Configurable Outport Control/1 -> Out1/1
  accumulation/1 -> Configurable Outport Control/1
  PTA Driver/2 -> PERIOD_COUNT/1
  PTA Driver/1 -> accumulation/1

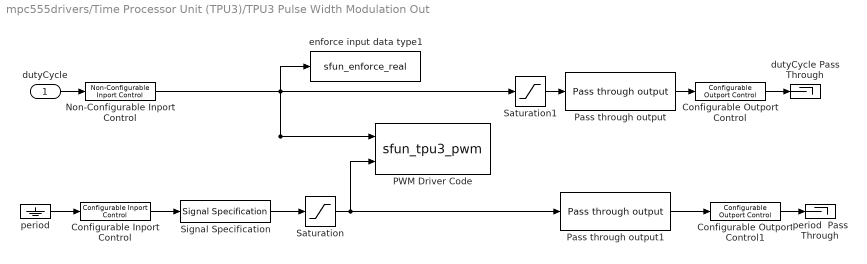
== system mpc555drivers/Time Processor Unit (TPU3)/TPU3 Pulse Width Modulation Out ==
  dutyCycle : Inport  Port=1  LatchInput=off
  Configurable Inport Control : passthrough/Configurable Inport Control  portNum=2  portName=Period  isEnabled=0  isConfigurable=1  isInport=1
  Configurable Outport Control : passthrough/Configurable Outport Control  portNum=1  portName=PassThroughDutyCycle  isEnabled=0  isConfigurable=1  isInport=0
  Configurable Outport Control1 : passthrough/Configurable Outport Control  portNum=2  portName=PassThroughPeriod  isEnabled=0  isConfigurable=1  isInport=0
  Non-Configurable Inport Control : passthrough/Non-Configurable Inport Control  portNum=1  isEnabled=1  isConfigurable=0  isInport=1
  PWM Driver Code : S-Function  FunctionName=sfun_tpu3_pwm  Parameters=sampleTime, module, uint8(channel), uint8(channel_priority), uint16(PWMPER), block_period
  Pass through output : passthrough/Pass through output  driverBlock=gcs
  Pass through output1 : passthrough/Pass through output  driverBlock=gcs
  Saturation : Saturate  UpperLimit=hex2dec('8000')  LowerLimit=0
  Saturation1 : Saturate  UpperLimit=1  LowerLimit=0
  Signal Specification : SignalSpecification  DataType=uint16
  dutyCycle Pass Through : Terminator
  enforce input data type1 : S-Function  FunctionName=sfun_enforce_real
  period : Ground
  period  Pass Through : Terminator
  wires:
  Saturation/1 -> Pass through output1/1, PWM Driver Code/2
  Saturation1/1 -> Pass through output/1
  Non-Configurable Inport Control/1 -> enforce input data type1/1, PWM Driver Code/1, Saturation1/1
  Signal Specification/1 -> Saturation/1
  Configurable Inport Control/1 -> Signal Specification/1
  Pass through output1/1 -> Configurable Outport Control1/1
  Pass through output/1 -> Configurable Outport Control/1
  Configurable Outport Control/1 -> dutyCycle Pass Through/1
  Configurable Outport Control1/1 -> period  Pass Through/1
  period/1 -> Configurable Inport Control/1
  dutyCycle/1 -> Non-Configurable Inport Control/1

== system mpc555drivers/Enhanced Queued Analog-To-Digital Converter Module-64/QADCE Analog In/Subsystem ==
  In1 : Inport  Port=1  LatchInput=off
  Data Type Conversion2 : DataTypeConversion  Tag=type_block  OutDataTypeMode=uint16  RndMeth=Zero
  Out1 : Outport
  wires:
  In1/1 -> Data Type Conversion2/1
  Data Type Conversion2/1 -> Out1/1

== system mpc555drivers/Execution Profiling/MPC555 Execution Profiling via CAN A/Send data over CAN ==
  In1 : Inport  Port=1  LatchInput=off
  Enable : EnablePort
  CAN Message Packing : canblocks/CAN Message Packing  id=dataId  message_type=Extended (29-bit identifier)  endian=Big Endian (Motorola)
  TouCAN Transmit : mpc555toucan/TouCAN Transmit  module=A  tx_mode=FIFO queued transmission with dedicated buffer  fifo_queue_length=8  bufferids=0  t=-1  enablePassThru=off
  wires:
  CAN Message Packing/1 -> TouCAN Transmit/1
  In1/1 -> CAN Message Packing/1

== system mpc555drivers/Execution Profiling/MPC555 Execution Profiling via CAN A/Start execution profiling ==
  function : TriggerPort  TriggerType=function-call  ZeroCross=off
  Execution Profiling Start : exprofilelib/Execution Profiling Start

== system mpc555drivers/Execution Profiling/MPC555 Execution Profiling via SCI1/Send Execution Profiling Data via Serial ==
  Enable : EnablePort
  Execution Profiling Output Data : exprofilelib/Execution Profiling Output Data  t=t
  Send data over serial : Subsystem  TreatAsAtomicUnit=on  PropExecContextAcrossSSBoundary=on
  wires:
  Execution Profiling Output Data/2 -> Send data over serial/1(In1)
  Execution Profiling Output Data/1 -> Send data over serial/Enable

== system mpc555drivers/Execution Profiling/MPC555 Execution Profiling via SCI1/Start Profiling ==
  Data In : Inport  Port=1  LatchInput=off
  Enable : EnablePort
  Recognise Start Byte : simulink/Logic and Bit Operations/Compare To Constant  relop===  const=201  LogicOutDataTypeMode=uint8
  Start execution profiling : Subsystem  PropExecContextAcrossSSBoundary=on
  wires:
  Recognise Start Byte/1 -> Start execution profiling/Enable
  Data In/1 -> Recognise Start Byte/1

== system mpc555drivers/Modular Input/Output System (MIOS1)/MIOS Digital In/Process Simulation Input ==
  SimIn : Inport  Port=1  LatchInput=off
  Constant : Constant  Value=0
  Data Type Conversion1 : DataTypeConversion  SaturateOnIntegerOverflow=on  RndMeth=Zero
  Relational Operator : RelationalOperator  Operator=>  LogicOutDataTypeMode=Boolean  InputSameDT=on
  SimOut : Outport
  wires:
  Constant/1 -> Data Type Conversion1/1
  Relational Operator/1 -> SimOut/1
  Data Type Conversion1/1 -> Relational Operator/2
  SimIn/1 -> Relational Operator/1

== system mpc555drivers/Modular Input/Output System (MIOS1)/MIOS Digital Out/Subsystem ==
  u : Inport  Port=1  LatchInput=off
  Disable MPC555 Interrupts : mpc555extras/Disable MPC555 Interrupts  Tag=Disable MPC555 Interrupts
  fd : Subsystem  TreatAsAtomicUnit=on  PropExecContextAcrossSSBoundary=on
  wires:
  u/1 -> fd/1(u)

== system mpc555drivers/Modular Input/Output System (MIOS1)/MIOS Waveform Measurement/Separate Signals ==
  AB : Inport  Port=1  LatchInput=off
  Bitwise Operator1 : mpc555extras/Bitwise Operator  logicop=SHIFT RIGHT  zeroTest=No Test  UseBitMask=on  BitMask=16  maskInBinary=off
  Bitwise Operator2 : mpc555extras/Bitwise Operator  logicop=AND  zeroTest=No Test  UseBitMask=on  BitMask='ffff'  maskInBinary=off
  Data Type Conversion1 : DataTypeConversion  OutDataTypeMode=uint16  RndMeth=Zero
  Data Type Conversion2 : DataTypeConversion  OutDataTypeMode=uint16  RndMeth=Zero
  A : Outport
  B : Outport  Port=2
  wires:
  AB/1 -> Bitwise Operator1/1, Bitwise Operator2/1
  Bitwise Operator1/1 -> Data Type Conversion1/1
  Bitwise Operator2/1 -> Data Type Conversion2/1
  Data Type Conversion1/1 -> A/1
  Data Type Conversion2/1 -> B/1

== system mpc555drivers/Queued Analog-To-Digital Converter Module-64/QADC Analog In/Process Simulation Input ==
  note: This subsystem implements appropriate scaling of the pass-through signal depending
      | on whether the QADC is set to right or left justfied, signed or unsigned.
  SimIn : Inport  Port=1  PortDimensions=num_channels  LatchInput=off
  Bitwise Operator : mpc555extras/Bitwise Operator  logicop=SHIFT LEFT  zeroTest=No Test  UseBitMask=on  BitMask=6  maskInBinary=off
  Constant : Constant  Value=justification
  Data Type Conversion : DataTypeConversion  OutDataTypeMode=uint16  SaturateOnIntegerOverflow=on  RndMeth=Zero
  Gain : Gain  Gain=2^10 - 1  SaturateOnIntegerOverflow=on
  Multiport Switch : MultiPortSwitch  Inputs=3  InputSameDT=on
  Saturation : Saturate  UpperLimit=1  LowerLimit=0  ZeroCross=off
  Switch Case Action Subsystem2 : Subsystem  AncestorBlock=|  PropExecContextAcrossSSBoundary=on
      | mpc555drivers/Queued
      | Analog-To-Digital
      | Converter Module-64/QADC Analog In
      | (Continuous-scan)/Switch Case Action
      | Subsystem1
  SimOut : Outport
  wires:
  Gain/1 -> Data Type Conversion/1
  Saturation/1 -> Gain/1
  Constant/1 -> Multiport Switch/1
  Bitwise Operator/1 -> Multiport Switch/3
  Switch Case Action Subsystem2/1(Out1) -> Multiport Switch/4
  Multiport Switch/1 -> SimOut/1
  SimIn/1 -> Saturation/1
  Data Type Conversion/1 -> Switch Case Action Subsystem2/1(In1), Multiport Switch/2, Bitwise Operator/1

== system mpc555drivers/Queued Analog-To-Digital Converter Module-64/QADC Analog In/Subsystem ==
  In1 : Inport  Port=1  LatchInput=off
  Data Type Conversion2 : DataTypeConversion  Tag=type_block  OutDataTypeMode=uint16  RndMeth=Zero
  Out1 : Outport
  wires:
  Data Type Conversion2/1 -> Out1/1
  In1/1 -> Data Type Conversion2/1

== system mpc555drivers/Queued Analog-To-Digital Converter Module-64/QADC Digital In/Process Simulation Input ==
  SimIn : Inport  Port=1  LatchInput=off
  Constant : Constant  Value=0
  Data Type Conversion : DataTypeConversion  OutDataTypeMode=boolean  SaturateOnIntegerOverflow=on  RndMeth=Zero
  Data Type Conversion1 : DataTypeConversion  SaturateOnIntegerOverflow=on  RndMeth=Zero
  Relational Operator : RelationalOperator  Operator=>  InputSameDT=on
  SimOut : Outport
  wires:
  Constant/1 -> Data Type Conversion1/1
  Relational Operator/1 -> Data Type Conversion/1
  Data Type Conversion1/1 -> Relational Operator/2
  Data Type Conversion/1 -> SimOut/1
  SimIn/1 -> Relational Operator/1
